simulink model "DPT_with_friction"  (R2023a)
settings: Solver=ode15s  StartTime=0.0  StopTime=1  RelTol=1e-3
settings Model: Creator=ПК  LastModifiedBy=ПК

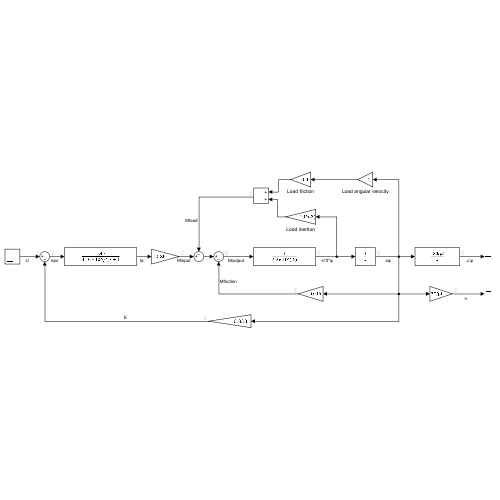
[thumbnail: Simulink's stored preview of the top-level diagram]
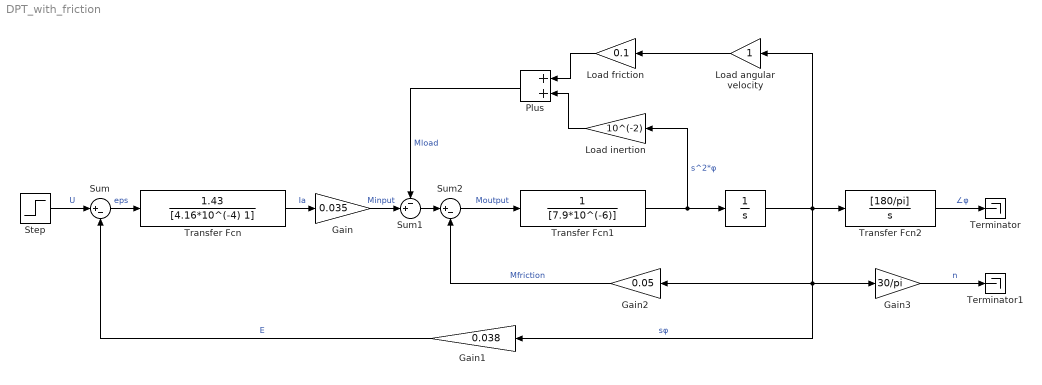
== system DPT_with_friction ==
  " " : TransferFcn  Denominator=[1 0]
  Gain : Gain  Gain=0.035
  Gain1 : Gain  Gain=0.038
  Gain2 : Gain  Gain=0.05
  Gain3 : Gain  Gain=30/pi
  Load angular velocity : Gain
  Load friction : Gain  Gain=0.1
  Load inertion : Gain  Gain=10^(-2)
  Plus : Sum
  Step : Step  Time=0  After=27  SampleTime=0
  Sum : Sum  Inputs=|+-
  Sum1 : Sum  Inputs=-+|
  Sum2 : Sum  Inputs=|+-
  Terminator : Terminator
  Terminator1 : Terminator
  Transfer Fcn : TransferFcn  Numerator=[1.43]  Denominator=[4.16*10^(-4) 1]
  Transfer Fcn1 : TransferFcn  Denominator=[7.9*10^(-6)]
  Transfer Fcn2 : TransferFcn  Numerator=[180/pi]  Denominator=[1 0]
  wires:
  Sum/1 -> Transfer Fcn/1  "eps"
  Transfer Fcn/1 -> Gain/1  "Ia"
  " "/1 -> Transfer Fcn2/1, Gain3/1, Gain1/1, Gain2/1, Load angular velocity/1  "sφ"
  Gain1/1 -> Sum/2  "E"
  Step/1 -> Sum/1  "U"
  Gain/1 -> Sum1/2  "Мinput"
  Transfer Fcn2/1 -> Terminator/1  "∠φ"
  Plus/1 -> Sum1/1  "Mload"
  Load friction/1 -> Plus/1
  Load inertion/1 -> Plus/2
  Load angular velocity/1 -> Load friction/1
  Sum1/1 -> Sum2/1
  Sum2/1 -> Transfer Fcn1/1  "Moutput"
  Transfer Fcn1/1 -> Load inertion/1, " "/1  "s^2*φ"
  Gain2/1 -> Sum2/2  "Mfriction"
  Gain3/1 -> Terminator1/1  "n"
